simulink library "ddc"  (Simulink 8.1)
settings: Solver=ode1  StartTime=0.0  StopTime=Inf  FixedStep=0.001  RelTol=1e-3
PostLoadFcn:
  | , if any(exist('dsrtsu_mdlpostloadfcn', 'file') == [2, 3, 6]), try dsrtsu_mdlpostloadfcn('Execute', bdroot); catch fprintf('Error in PostLoadFcn (dsrtsu_mdlpostloadfcn) for model "%s":\n %s\n', bdroot, lasterr); end, end,
undefined symbols (not defined in the file or in its folder): KACC_OffsetToBumper_m, KACC_StoppingDistSafety_m
settings Model: DSRTSU_INTERNAL_RTI_VER=450  DSRTSU_INTERNAL_RTI_TYPE=rti1401  RTICANMMDATA=struct('GeneralSetupData',struct('modelroot','D:\ELN150201_TAIWAN\trunk\AdasDragon\software\sw_development\arch\app\acc','generalsettings',struct('filesettings',struct('destfolder',struct('Name','RTICANMM_FILES','Check',1),'buildfolder',struct('Name','.','Check',1),'AbsDestfolder',struct('Name','D:\ELN150201_TAIWAN\trunk\AdasDragon\software\sw_development\arch\app\acc\RTICANMM_FILES'),'AbsBuildfolder',struct('Name','D:\ELN150201_TAIWAN\trunk\AdasDragon\software\sw_development\arch\app\acc'))),'options',struct('addpaths',1,'rmpaths',1,'addtrcexclusion',logical(1),'cannavigator',struct('checkmonitoring',0),'show_usrtrc',0,'use_usrtrc',0),'advanced',struct('options',[1 1 1 1 1 1 1 1 1 1 1 1 1 1 1 1 1 1 1 1 1 1 1 1 1 1 1 1 1 1 1 1 1 1 1 1 1 1 1 1 1 1 1 1 1 1 1 1 1 1 1 1 1 1 1 1 1 1 1 1 1 1 1 1 1 1 1 1 1 1 1 1 1 1 1 1 1 1 1 1 1 1 1 1 1 1 1 1 1 1 1 1 1 1 1 1 1 1 1 1]),'MPSetup',{{}},'modelname','ddc','block','ddc'))  DSRTSU_INTERNAL_RTIFPGA=40  Creator=AT015555  LastModifiedBy=AT015555

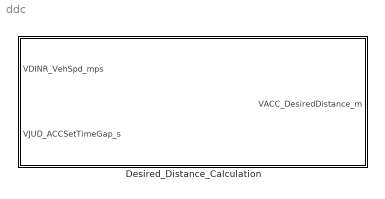
== system ddc ==
  Desired_Distance_Calculation : Subsystem

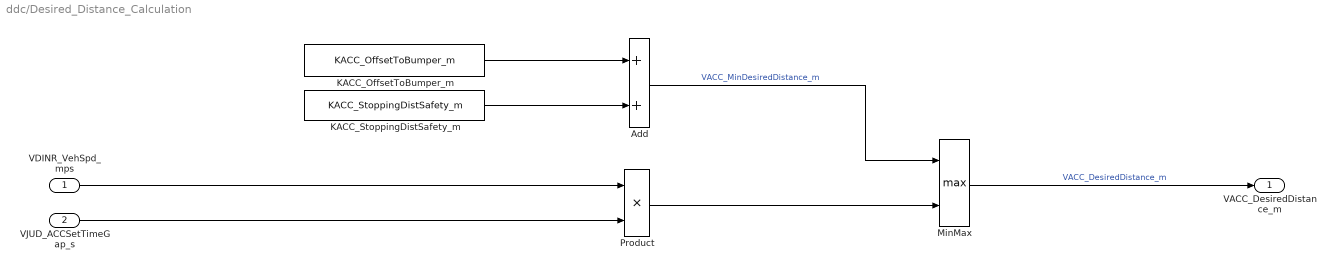
== system ddc/Desired_Distance_Calculation ==
  VDINR_VehSpd_mps : Inport
  VJUD_ACCSetTimeGap_s : Inport  Port=2
  Add : Sum
  KACC_OffsetToBumper_m : Constant  Value=KACC_OffsetToBumper_m
  KACC_StoppingDistSafety_m : Constant  Value=KACC_StoppingDistSafety_m
  MinMax : MinMax  Function=max  Inputs=2
  Product : Product
  VACC_DesiredDistance_m : Outport
  wires:
  Product/1 -> MinMax/2
  KACC_OffsetToBumper_m/1 -> Add/1
  MinMax/1 -> VACC_DesiredDistance_m/1  "VACC_DesiredDistance_m"
  KACC_StoppingDistSafety_m/1 -> Add/2
  VDINR_VehSpd_mps/1 -> Product/1
  Add/1 -> MinMax/1  "VACC_MinDesiredDistance_m"
  VJUD_ACCSetTimeGap_s/1 -> Product/2
